simulink model "inga3"  (Simulink 7.8)
settings: Solver=ode45  StartTime=0.0  StopTime=50  RelTol=1e-8
undefined symbols (not defined in the file or in its folder): x, xprime
libraries: vrlib x3
settings Model: Creator=valaki  ModifiedByFormat=Balazs  LastModifiedBy=Balazs
settings DataIOCC: SaveOutput=off  SignalLogging=off  SaveTime=off
settings OptimizationCC: InitFltsAndDblsToZero=on
settings DebuggingCC: SaveWithParameterizedLinksMsg=none  SignalResolutionControl=TryResolveAllWithWarning  SolverPrmCheckMsg=none  MultiTaskDSMMsg=warning  MultiTaskCondExecSysMsg=none  FcnCallInpInsideContextMsg=Use local settings  StrictBusMsg=Warning
settings RTWCC: IncludeERTFirstTime=on
settings GRTTargetCC: TargetFcnLib=ansi_tfl_tmw.mat

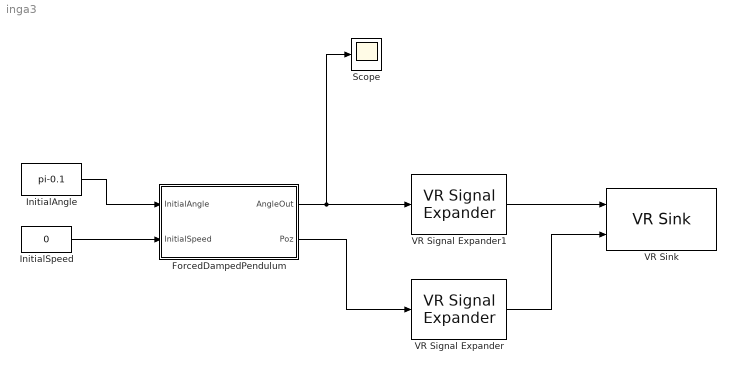
== system inga3 ==
  ForcedDampedPendulum : Subsystem
  InitialAngle : Constant  Value=pi-0.1
  InitialSpeed : Constant  Value=0
  Scope : Scope
      settings: YMin=-14  YMax=3
  VR Signal Expander : vrlib/VR Signal Expander  outwidth=3  outidx=[1]
  VR Signal Expander1 : vrlib/VR Signal Expander  outwidth=4  outidx=[ 4 ]
  VR Sink : vrlib/VR Sink  SampleTime=0.1  ViewEnable=on  RemoteChange=off  RemoteView=off  FieldsWritten=Ball.rotation.4.1.double#Ball.translation.3.1.double  WorldFileName=Pendulum_3D.wrl  WorldDescription=Forced Damped Pendulum  AutoView=off  VideoDimensions=[]  AllowVariableSize=off  FigureProperties="{'Position', 'Name', 'Viewpoint', 'CameraBound', 'CameraDirection', 'CameraPosition', 'CameraUpVector', 'ZoomFactor', 'Antialiasing', 'Headlight', 'Lighting', 'NavPanel', 'StatusBar', 'ToolBar', 'Textures', 'Transparency', 'Triad', 'Wireframe', 'NavZones', 'NavMode', 'NavSpeed', 'CaptureFileFormat', 'CaptureFileName', 'Record2DCompressMethod', 'Record2DCompressQuality', 'Record2D', 'Record2DFileName', 'Record2DFPS'; [5.0000000000000000e+000  9.2000000000000000e+001  5.7600000000000000e+002  3.8000000000000000e+002], 'Forced Damped Pendulum', 'Ball', 'on', [0.0000000000000000e+000  0.0000000000000000e+000 -1.0000000000000000e+000], [0.0000000000000000e+000  0.0000000000000000e+000  0.0000000000000000e+000], [0.0000000000000000e+000  1.0000000000000000e+000  0.0000000000000000e+000], [1.0000000000000000e+000], 'on', 'on', 'on', 'halfbar', 'on', 'on', 'on', 'on', 'none', 'off', 'off', 'fly', 'normal', 'tif', '%f_anim_%n.tif', 'auto', [7.5000000000000000e+001], 'off', '%f_anim_%n.avi', [1.5000000000000000e+001]}"
  wires:
  InitialAngle/1 -> ForcedDampedPendulum/1(InitialAngle)
  InitialSpeed/1 -> ForcedDampedPendulum/2(InitialSpeed)
  ForcedDampedPendulum/1(AngleOut) -> VR Signal Expander1/1, Scope/1
  VR Signal Expander1/1 -> VR Sink/1
  ForcedDampedPendulum/2(Poz) -> VR Signal Expander/1
  VR Signal Expander/1 -> VR Sink/2

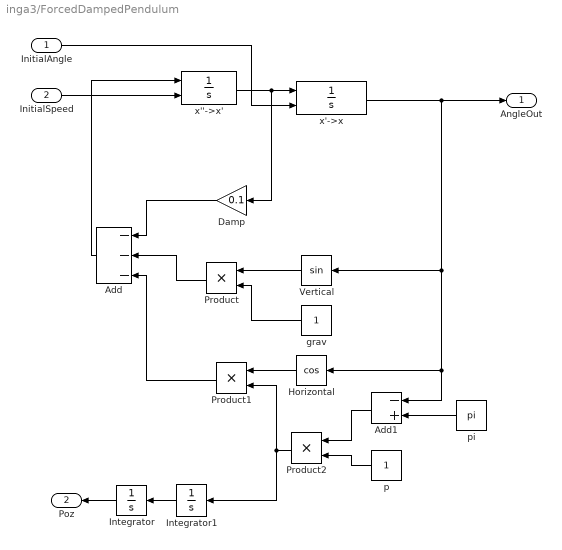
== system inga3/ForcedDampedPendulum ==
  InitialAngle : Inport
  InitialSpeed : Inport  Port=2
  Add : Sum  Inputs=---
  Add1 : Sum  Inputs=-+
  Damp : Gain  Gain=0.1
  Horizontal : Trigonometry  Operator=cos
  Integrator : Integrator
  Integrator1 : Integrator
  Product : Product  RndMeth=Zero
  Product1 : Product  RndMeth=Zero
  Product2 : Product  RndMeth=Zero
  Vertical : Trigonometry
  grav : Constant
  p : Constant
  pi : Constant  Value=pi
  x''->x' : Integrator  InitialConditionSource=external  InitialCondition=xprime
  x'->x : Integrator  InitialConditionSource=external  InitialCondition=x
  AngleOut : Outport
  Poz : Outport  Port=2
  wires:
  x'->x/1 -> AngleOut/1, Vertical/1, Horizontal/1, Add1/1
  x''->x'/1 -> Damp/1, x'->x/1
  Add/1 -> x''->x'/1
  Damp/1 -> Add/1
  InitialSpeed/1 -> x''->x'/2
  InitialAngle/1 -> x'->x/2
  Vertical/1 -> Product/1
  Product/1 -> Add/2
  Integrator1/1 -> Integrator/1
  Integrator/1 -> Poz/1
  grav/1 -> Product/2
  Horizontal/1 -> Product1/1
  p/1 -> Product2/2
  Product2/1 -> Product1/2, Integrator1/1
  Add1/1 -> Product2/1
  pi/1 -> Add1/2
  Product1/1 -> Add/3
